simulink model "katana_control"  (R2020a)
settings: Solver=ode8  StartTime=0.0  StopTime=20  FixedStep=0.004  MaxStep=0.004  RelTol=1e-3
InitFcn:
  | [lowpass_B, lowpass_A] = butter(4,1,'s');
  | manipulator_tree = importrobot('../../catkin_ws/src/katana_description/katana_description.urdf');
  | manipulator_tree.Gravity = [0 0 -9.81];
model workspace (MAT data in the model file):
  SL_ROS_VariableLengthArrays_MaxSizes.CommonInfo.ArrayTruncateAction = 'EmitWarning'
  SL_ROS_VariableLengthArrays_MaxSizes.MsgTypeMap = containers.Map
  SL_ROS_VariableLengthArrays_MaxSizes.MsgTypeMap.serialization.keys = {'std_msgs/Float32MultiArray', 'std_msgs/Float64MultiArray'}
  SL_ROS_VariableLengthArrays_MaxSizes.MsgTypeMap.serialization.values{1}.PropertyName = 'Data'
  SL_ROS_VariableLengthArrays_MaxSizes.MsgTypeMap.serialization.values{1}.DataType = 'single'
  SL_ROS_VariableLengthArrays_MaxSizes.MsgTypeMap.serialization.values{1}.MaxLength = 14
  SL_ROS_VariableLengthArrays_MaxSizes.MsgTypeMap.serialization.values{2}.PropertyName = 'Data'
  SL_ROS_VariableLengthArrays_MaxSizes.MsgTypeMap.serialization.values{2}.DataType = 'double'
  SL_ROS_VariableLengthArrays_MaxSizes.MsgTypeMap.serialization.values{2}.MaxLength = 7
  SL_ROS_VariableLengthArrays_MaxSizes.MsgTypeMap.serialization.uniformity = 0
  SL_ROS_VariableLengthArrays_MaxSizes.MsgTypeMap.serialization.keyType = 'char'
  SL_ROS_VariableLengthArrays_MaxSizes.MsgTypeMap.serialization.valueType = 'any'
undefined symbols (not defined in the file or in its folder): Data, Data_SL_Info
libraries: robotlib x11, robotmaniplib x1
settings Model: Creator=marco  LastModifiedBy=marco
settings OptimizationCC: EnhancedBackFolding=on  PassReuseOutputArgsAs=Individual arguments  ZeroExternalMemoryAtStartup=off  ZeroInternalMemoryAtStartup=off  MaxStackSize=64  OptimizeBlockOrder=speed  DifferentSizesBufferReuse=on  OptimizationCustomize=off  EfficientTunableParamExpr=on
settings DebuggingCC: ParameterTunabilityLossMsg=error
settings HardwareCC: ProdBitPerLong=64  ProdHWDeviceType=Intel->x86-64 (Linux 64)
settings RTWCC: SystemTargetFile=ert.tlc  HardwareBoard=Robot Operating System (ROS)  TemplateMakefile=ert_default_tmf  Toolchain=Catkin  TargetLang=C++
settings CodeAppCC: ForceParamTrailComments=on  IgnoreCustomStorageClasses=off  OperatorAnnotations=on  SimulinkDataObjDesc=on  SFDataObjDesc=on  InsertBlockDesc=on
settings ERTTargetCC: SupportContinuousTime=on  SupportVariableSizeSignals=on

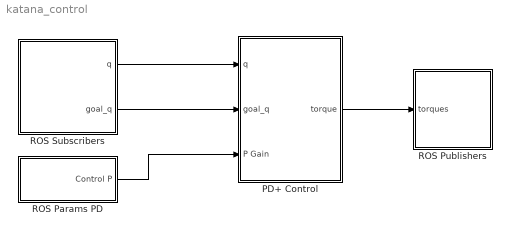
== system katana_control ==
  PD+ Control : Subsystem
  ROS Params PD : Subsystem
  ROS Publishers : Subsystem
  ROS Subscribers : Subsystem
  wires:
  PD+ Control/1(torque) -> ROS Publishers/1(torques)
  ROS Subscribers/2(goal_q) -> PD+ Control/2(goal_q)
  ROS Subscribers/1(q) -> PD+ Control/1(q)
  ROS Params PD/1(Control P) -> PD+ Control/3(P Gain)

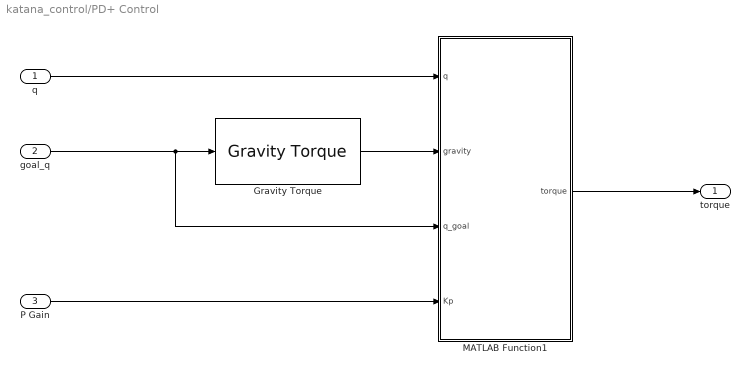
== system katana_control/PD+ Control ==
  q : Inport
  goal_q : Inport  Port=2
  P Gain : Inport  Port=3
  Gravity Torque : robotmaniplib/Gravity Torque  RigidBodyTree=manipulator_tree  SimulateUsing=Code generation
  MATLAB Function1 : MATLAB Function  TreatAsAtomicUnit=on
  torque : Outport
  wires:
  P Gain/1 -> MATLAB Function1/4(Kp)
  q/1 -> MATLAB Function1/1(q)
  goal_q/1 -> Gravity Torque/1, MATLAB Function1/3(q_goal)
  MATLAB Function1/1(torque) -> torque/1
  Gravity Torque/1 -> MATLAB Function1/2(gravity)

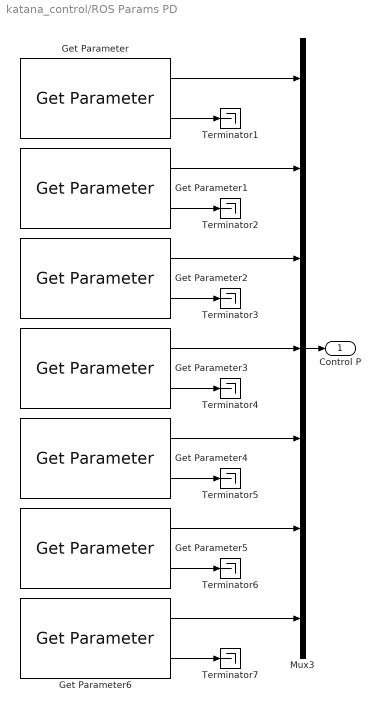
== system katana_control/ROS Params PD ==
  Get Parameter : robotlib/Get Parameter  ParameterSource=Specify your own  ParameterName=/control/P1  ParameterType=double  ParameterMaxArrayLength=16  ParameterInitialValue=0.0  SampleTime=1  ShowErrorCodeOutput=on  ModelName=katana_control  BlockId=ParamGet_katana_control_343
      settings: SourceProductBaseCode=RR
  Get Parameter1 : robotlib/Get Parameter  ParameterSource=Specify your own  ParameterName=/control/P2  ParameterType=double  ParameterMaxArrayLength=16  ParameterInitialValue=0.0  SampleTime=1  ShowErrorCodeOutput=on  ModelName=katana_control  BlockId=ParamGet_katana_control_344
      settings: SourceProductBaseCode=RR
  Get Parameter2 : robotlib/Get Parameter  ParameterSource=Specify your own  ParameterName=/control/P3  ParameterType=double  ParameterMaxArrayLength=16  ParameterInitialValue=0.0  SampleTime=1  ShowErrorCodeOutput=on  ModelName=katana_control  BlockId=ParamGet_katana_control_349
      settings: SourceProductBaseCode=RR
  Get Parameter3 : robotlib/Get Parameter  ParameterSource=Specify your own  ParameterName=/control/P4  ParameterType=double  ParameterMaxArrayLength=16  ParameterInitialValue=0.0  SampleTime=1  ShowErrorCodeOutput=on  ModelName=katana_control  BlockId=ParamGet_katana_control_350
      settings: SourceProductBaseCode=RR
  Get Parameter4 : robotlib/Get Parameter  ParameterSource=Specify your own  ParameterName=/control/P5  ParameterType=double  ParameterMaxArrayLength=16  ParameterInitialValue=0.0  SampleTime=1  ShowErrorCodeOutput=on  ModelName=katana_control  BlockId=ParamGet_katana_control_351
      settings: SourceProductBaseCode=RR
  Get Parameter5 : robotlib/Get Parameter  ParameterSource=Specify your own  ParameterName=/control/P6  ParameterType=double  ParameterMaxArrayLength=16  ParameterInitialValue=0.0  SampleTime=1  ShowErrorCodeOutput=on  ModelName=katana_control  BlockId=ParamGet_katana_control_352
      settings: SourceProductBaseCode=RR
  Get Parameter6 : robotlib/Get Parameter  ParameterSource=Specify your own  ParameterName=/control/P7  ParameterType=double  ParameterMaxArrayLength=16  ParameterInitialValue=0.0  SampleTime=1  ShowErrorCodeOutput=on  ModelName=katana_control  BlockId=ParamGet_katana_control_353
      settings: SourceProductBaseCode=RR
  Mux3 : Mux  Inputs=7
  Terminator{1..7} (7 alike) : Terminator
  Control P : Outport
  wires:
  Get Parameter5/1 -> Mux3/6
  Get Parameter2/1 -> Mux3/3
  Get Parameter/1 -> Mux3/1
  Get Parameter3/1 -> Mux3/4
  Get Parameter/2 -> Terminator1/1
  Get Parameter4/1 -> Mux3/5
  Get Parameter6/2 -> Terminator7/1
  Get Parameter6/1 -> Mux3/7
  Get Parameter2/2 -> Terminator3/1
  Get Parameter1/2 -> Terminator2/1
  Get Parameter5/2 -> Terminator6/1
  Get Parameter1/1 -> Mux3/2
  Get Parameter4/2 -> Terminator5/1
  Get Parameter3/2 -> Terminator4/1
  Mux3/1 -> Control P/1

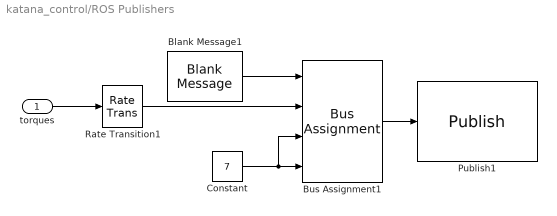
== system katana_control/ROS Publishers ==
  torques : Inport
  Blank Message1 : robotlib/Blank Message  messageClass=Message  entityType=std_msgs/Float64MultiArray  messageType=std_msgs/Float64MultiArray  SampleTime=0.004
  Bus Assignment1 : BusAssignment  AssignedSignals=Data,Data_SL_Info.CurrentLength,Data_SL_Info.ReceivedLength
  Constant : Constant  Value=7  OutDataTypeStr=uint32  SampleTime=0.004
  Publish1 : robotlib/Publish  topicSource=Specify your own  topic=/joint_torques  messageType=std_msgs/Float64MultiArray  messageQueueLength=1
  Rate Transition1 : RateTransition
  wires:
  Blank Message1/1 -> Bus Assignment1/1
  Rate Transition1/1 -> Bus Assignment1/2
  torques/1 -> Rate Transition1/1
  Bus Assignment1/1 -> Publish1/1
  Constant/1 -> Bus Assignment1/4, Bus Assignment1/3

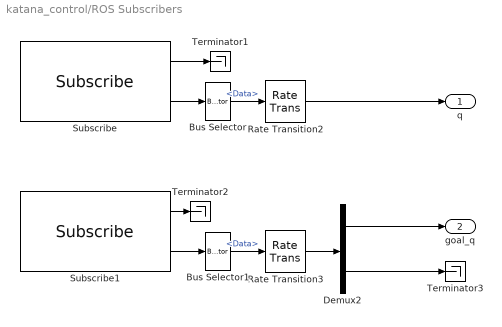
== system katana_control/ROS Subscribers ==
  Bus Selector : BusSelector  OutputSignals=Data
  Bus Selector1 : BusSelector  OutputSignals=Data
  Demux2 : Demux  Outputs=[7,7]
  Rate Transition2 : RateTransition
  Rate Transition3 : RateTransition
  Subscribe : robotlib/Subscribe  topicSource=Specify your own  topic=/joint_positions  messageType=std_msgs/Float64MultiArray  sampleTime=0.004  messageQueueLength=1
  Subscribe1 : robotlib/Subscribe  topicSource=Specify your own  topic=/goal_trajectory  messageType=std_msgs/Float32MultiArray  sampleTime=0.004  messageQueueLength=1
  Terminator1 : Terminator
  Terminator2 : Terminator
  Terminator3 : Terminator
  q : Outport
  goal_q : Outport  Port=2
  wires:
  Subscribe1/1 -> Terminator2/1
  Subscribe1/2 -> Bus Selector1/1
  Bus Selector/1 -> Rate Transition2/1  "<Data>"
  Rate Transition2/1 -> q/1
  Demux2/1 -> goal_q/1
  Subscribe/2 -> Bus Selector/1
  Rate Transition3/1 -> Demux2/1
  Demux2/2 -> Terminator3/1
  Bus Selector1/1 -> Rate Transition3/1  "<Data>"
  Subscribe/1 -> Terminator1/1

== matlab function katana_control/PD+ Control/MATLAB Function1 ==
  data: q input; gravity input; q_goal input; torque output; Kp input
function torque = position_control(q,gravity, q_goal, Kp)
%%Constantes del control PD

qe = zeros(7,1);
torque = zeros(7,1);
for i=1:7
    qe(i) = q_goal(i) - q(i);
    torque(i) = gravity(i) + Kp(i)*qe(i);
end
